simulink model "StepperMotorController"  (Simulink 8.5)
settings: Solver=ode45  StartTime=0.0  StopTime=20  RelTol=1e-3
values from neighbouring files (symbols this model uses):
  brakegapIC = 25    [brakingTrajectory.m]
settings Model: Creator=MrPiccolo  LastModifiedBy=MrPiccolo
settings DataIOCC: SignalLoggingSaveFormat=Dataset
settings OptimizationCC: ExpressionDepthLimit=128
settings DebuggingCC: UnderspecifiedInitializationDetection=Simplified  MergeDetectMultiDrivingBlocksExec=error  FcnCallInpInsideContextMsg=EnableAllAsError  StateNameClashWarn=none
settings GRTTargetCC: CombineOutputUpdateFcns=on  GRTInterface=off

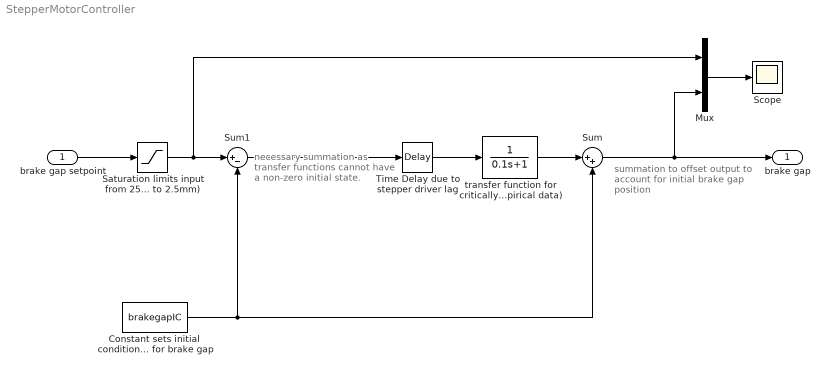
== system StepperMotorController ==
  note: necessary summation
      | as transfer functions
      | cannot have a
      | non-zero initial state.
  note: summation to offset
      | output to account for
      | initial brake gap position
  brake gap setpoint : Inport
  Constant sets initial  condition for brake gap : Constant  Value=brakegapIC
  Mux : Mux  Inputs=2
  Saturation limits input from 25mm to 2.5mm) : Saturate  UpperLimit=25  LowerLimit=2.5
  Scope : Scope
      settings: TimeRange=20  YMin=0  YMax=1.5
  Sum : Sum  Inputs=|++
  Sum1 : Sum  Inputs=|+-
  Time Delay due to stepper driver lag : TransportDelay  DelayTime=.05
  transfer function for critically damped 1st order system (this TF is intended to describe stepper motor response dynamics - should be validated  with empirical data) : TransferFcn  Denominator=[0.1 1]
  brake gap : Outport
  wires:
  Mux/1 -> Scope/1
  brake gap setpoint/1 -> Saturation limits input from 25mm to 2.5mm)/1
  Saturation limits input from 25mm to 2.5mm)/1 -> Mux/1, Sum1/1
  Sum/1 -> brake gap/1, Mux/2
  Time Delay due to stepper driver lag/1 -> transfer function for critically damped 1st order system (this TF is intended to describe stepper motor response dynamics - should be validated  with empirical data)/1
  Constant sets initial  condition for brake gap/1 -> Sum/2, Sum1/2
  transfer function for critically damped 1st order system (this TF is intended to describe stepper motor response dynamics - should be validated  with empirical data)/1 -> Sum/1
  Sum1/1 -> Time Delay due to stepper driver lag/1
